simulink model "gm_NRPolarDecodeHDL"  (R2020a)
settings: Solver=FixedStepDiscrete  StartTime=0.0  StopTime=simTime  RelTol=1e-3
undefined symbols (not defined in the file or in its folder): sampleTime
libraries: dspsrcs4 x4, whdledac x1, whdlutilities x1
settings Model: Creator=The MathWorks, Inc.  LastModifiedBy=joys_mbuku
settings OptimizationCC: BlockReduction=off  ConditionallyExecuteInputs=off  DefaultParameterBehavior=Inlined
settings DebuggingCC: AlgebraicLoopMsg=error  InheritedTsInSrcMsg=none  SingleTaskRateTransMsg=error
settings HardwareCC: ProdBitPerPointer=32  ProdBitPerSizeT=32  ProdBitPerPtrDiffT=32  ProdLargestAtomicFloat=None  ProdIntDivRoundTo=Undefined  ProdEndianess=Unspecified  ProdWordSize=32  ProdHWDeviceType=ASIC/FPGA->ASIC/FPGA  TargetBitPerPointer=64  TargetBitPerSizeT=64  TargetBitPerPtrDiffT=64  TargetLongLongMode=on  TargetIntDivRoundTo=Zero  TargetEndianess=LittleEndian  TargetWordSize=64  TargetHWDeviceType=Custom Processor->MATLAB Host Computer  ProdEqTarget=off

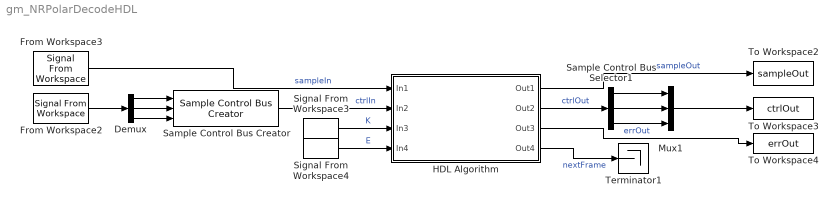
== system gm_NRPolarDecodeHDL ==
  Demux : Demux  Outputs=3
  From Workspace2 : dspsrcs4/Signal From Workspace  X=decCtrlIn  Ts=sampleTime  nsamps=1  OutputAfterFinalValue=Setting to zero  ignoreOrWarnInputAndFrameLengths=off  OutputFrames=off
  From Workspace3 : dspsrcs4/Signal From Workspace  X=decSampleIn  Ts=sampleTime  nsamps=1  OutputAfterFinalValue=Setting to zero  ignoreOrWarnInputAndFrameLengths=off  OutputFrames=off
  HDL Algorithm : Subsystem
  Mux1 : Mux  Inputs=3
  Sample Control Bus Creator : whdlutilities/Sample Control Bus Creator
      settings: SourceProductBaseCode=LH
  Sample Control Bus Selector1 : BusSelector  OutputSignals=start,end,valid
  Signal From Workspace3 : dspsrcs4/Signal From Workspace  X=decKfi  Ts=sampleTime  nsamps=1  OutputAfterFinalValue=Setting to zero  ignoreOrWarnInputAndFrameLengths=off  OutputFrames=off
  Signal From Workspace4 : dspsrcs4/Signal From Workspace  X=decEfi  Ts=sampleTime  nsamps=1  OutputAfterFinalValue=Setting to zero  ignoreOrWarnInputAndFrameLengths=off  OutputFrames=off
  Terminator1 : Terminator
  To Workspace2 : ToWorkspace  VariableName=sampleOut  SampleTime=-1
      settings: MaxDataPoints=simTime  Save2DSignal=2-D array (concatenate along first dimension)
  To Workspace3 : ToWorkspace  VariableName=ctrlOut  SampleTime=-1
      settings: MaxDataPoints=simTime  Save2DSignal=2-D array (concatenate along first dimension)
  To Workspace4 : ToWorkspace  VariableName=errOut  SampleTime=-1
      settings: MaxDataPoints=simTime  Save2DSignal=2-D array (concatenate along first dimension)
  wires:
  HDL Algorithm/4(Out4) -> Terminator1/1  "nextFrame"
  HDL Algorithm/3(Out3) -> To Workspace4/1  "errOut"
  HDL Algorithm/2(Out2) -> Sample Control Bus Selector1/1  "ctrlOut"
  HDL Algorithm/1(Out1) -> To Workspace2/1  "sampleOut"
  Signal From Workspace4/1 -> HDL Algorithm/4(In4)  "E"
  Signal From Workspace3/1 -> HDL Algorithm/3(In3)  "K"
  Sample Control Bus Creator/1 -> HDL Algorithm/2(In2)  "ctrlIn"
  From Workspace3/1 -> HDL Algorithm/1(In1)  "sampleIn"
  Demux/1 -> Sample Control Bus Creator/1
  Demux/2 -> Sample Control Bus Creator/2
  Demux/3 -> Sample Control Bus Creator/3
  From Workspace2/1 -> Demux/1
  Sample Control Bus Selector1/3 -> Mux1/3
  Sample Control Bus Selector1/2 -> Mux1/2
  Sample Control Bus Selector1/1 -> Mux1/1
  Mux1/1 -> To Workspace3/1

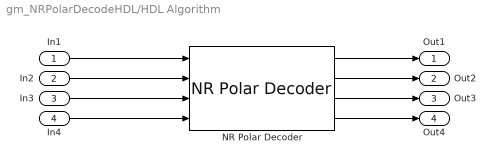
== system gm_NRPolarDecodeHDL/HDL Algorithm ==
  In1 : Inport
  In2 : Inport  Port=2
  In3 : Inport  Port=3
  In4 : Inport  Port=4
  NR Polar Decoder : whdledac/NR Polar Decoder  LinkDirection=Uplink  ConfigurationSource=Input port  MessageLength=K  Rate=864  RNTIPort=off  DebugPortsEn=0  SimulateUsing=Code generation
      settings: SourceProductBaseCode=LH
  Out1 : Outport
  Out2 : Outport  Port=2
  Out3 : Outport  Port=3
  Out4 : Outport  Port=4
  wires:
  In1/1 -> NR Polar Decoder/1
  In4/1 -> NR Polar Decoder/4
  NR Polar Decoder/1 -> Out1/1
  NR Polar Decoder/4 -> Out4/1
  In2/1 -> NR Polar Decoder/2
  NR Polar Decoder/2 -> Out2/1
  NR Polar Decoder/3 -> Out3/1
  In3/1 -> NR Polar Decoder/3
